simulink model "sistemasRetroalimentadosSimulaciones"  (R2019a)
settings: Solver=VariableStepAuto  StartTime=0.0  StopTime=100  RelTol=1e-3
settings Model: Creator=pon_c  LastModifiedBy=pon_c

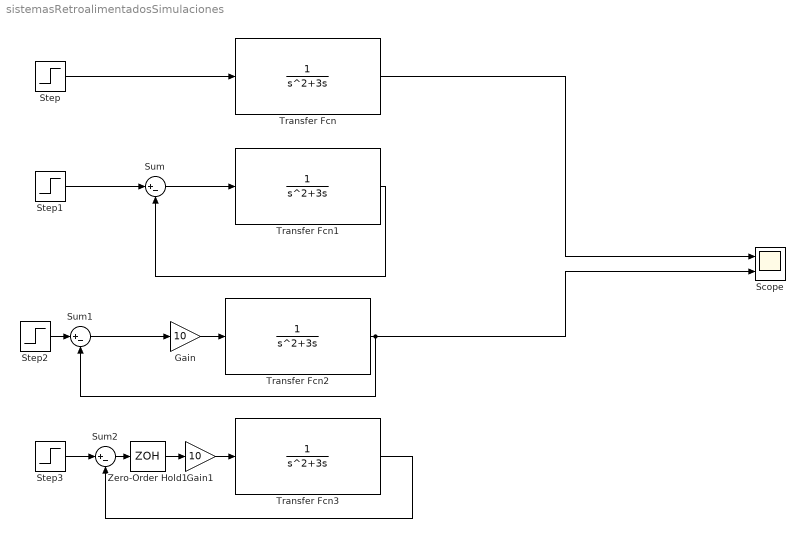
== system sistemasRetroalimentadosSimulaciones ==
  Gain : Gain  Gain=10
  Gain1 : Gain  Gain=10
  Scope : Scope  NumInputPorts=2
  Step{,1..3} (4 alike) : Step  SampleTime=0
  Sum : Sum  Inputs=|+-
  Sum1 : Sum  Inputs=|+-
  Sum2 : Sum  Inputs=|+-
  Transfer Fcn{,1..3} (4 alike) : TransferFcn  Denominator=[1 3 0]
  Zero-Order Hold1 : ZeroOrderHold  SampleTime=100
  wires:
  Step/1 -> Transfer Fcn/1
  Transfer Fcn/1 -> Scope/1
  Step1/1 -> Sum/1
  Transfer Fcn1/1 -> Sum/2
  Sum/1 -> Transfer Fcn1/1
  Step2/1 -> Sum1/1
  Gain/1 -> Transfer Fcn2/1
  Zero-Order Hold1/1 -> Gain1/1
  Transfer Fcn3/1 -> Sum2/2
  Sum2/1 -> Zero-Order Hold1/1
  Step3/1 -> Sum2/1
  Gain1/1 -> Transfer Fcn3/1
  Sum1/1 -> Gain/1
  Transfer Fcn2/1 -> Sum1/2, Scope/2
